simulink model "einfacher_Prozess_Zustandsregler"  (Simulink 7.5)
settings: Solver=ode45  StartTime=0.0  StopTime=10.0  RelTol=1e-3
values from neighbouring files (symbols this model uses):
  KV = KV'    [Reglerauslegung.m]    (also in Test_Reglerauslegung.m; auslegung.m)
undefined symbols (not defined in the file or in its folder): KR1, KR2, KR3, MU1, MU2, MU3
settings Model: Creator=Mattse  LastModifiedBy=Mattse
settings DebuggingCC: FcnCallInpInsideContextMsg=Enable All

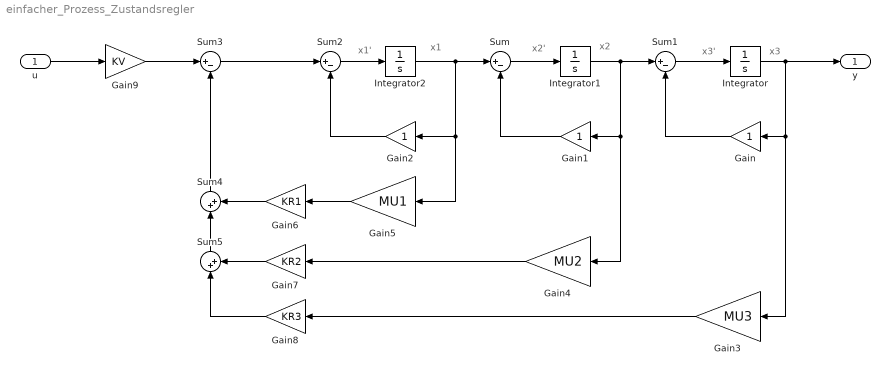
== system einfacher_Prozess_Zustandsregler ==
  note: x1'
  note: x1
  note: x2'
  note: x2
  note: x3'
  note: x3
  u : Inport
  Gain : Gain
  Gain1 : Gain
  Gain2 : Gain
  Gain3 : Gain  Gain=MU3
  Gain4 : Gain  Gain=MU2
  Gain5 : Gain  Gain=MU1
  Gain6 : Gain  Gain=KR1
  Gain7 : Gain  Gain=KR2
  Gain8 : Gain  Gain=KR3
  Gain9 : Gain  Gain=KV
  Integrator : Integrator
  Integrator1 : Integrator
  Integrator2 : Integrator
  Sum{,1..3} (4 alike) : Sum  Inputs=|+-
  Sum4 : Sum  Inputs=|++
  Sum5 : Sum  Inputs=|++
  y : Outport
  wires:
  Integrator1/1 -> Sum1/1, Gain1/1, Gain4/1
  Sum1/1 -> Integrator/1
  Sum/1 -> Integrator1/1
  Integrator2/1 -> Sum/1, Gain2/1, Gain5/1
  Sum2/1 -> Integrator2/1
  Integrator/1 -> y/1, Gain/1, Gain3/1
  Gain/1 -> Sum1/2
  Gain1/1 -> Sum/2
  Gain2/1 -> Sum2/2
  Sum3/1 -> Sum2/1
  Gain6/1 -> Sum4/2
  Gain5/1 -> Gain6/1
  Gain4/1 -> Gain7/1
  Gain3/1 -> Gain8/1
  Gain8/1 -> Sum5/1
  Gain7/1 -> Sum5/2
  Sum5/1 -> Sum4/1
  Sum4/1 -> Sum3/2
  u/1 -> Gain9/1
  Gain9/1 -> Sum3/1
